simulink model "jenkins_simulink_model"  (R2021a)
settings: Solver=VariableStepAuto  StartTime=0.0  StopTime=10  RelTol=1e-3
libraries: simulink x1
settings Model: Creator=PC  LastModifiedBy=PC

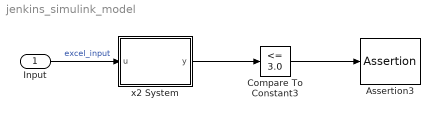
== system jenkins_simulink_model ==
  Input : Inport
  Assertion3 : Assertion
  Compare To Constant3 : simulink/Logic and Bit Operations/Compare To Constant  relop=<=  const=3.0  OutDataTypeStr=boolean
  x2 System : MATLAB Function  TreatAsAtomicUnit=on
  wires:
  Compare To Constant3/1 -> Assertion3/1
  Input/1 -> x2 System/1(u)  "excel_input"
  x2 System/1(y) -> Compare To Constant3/1

== matlab function jenkins_simulink_model/x2 System ==
  data: u input; y output
function y = fcn(u)
y = 2*u;
